simulink model "SINWave"  (R2023a)
settings: Solver=VariableStepAuto  StartTime=0.0  StopTime=10.0  RelTol=1e-3
settings Model: Creator=Lenovo  LastModifiedBy=Lenovo

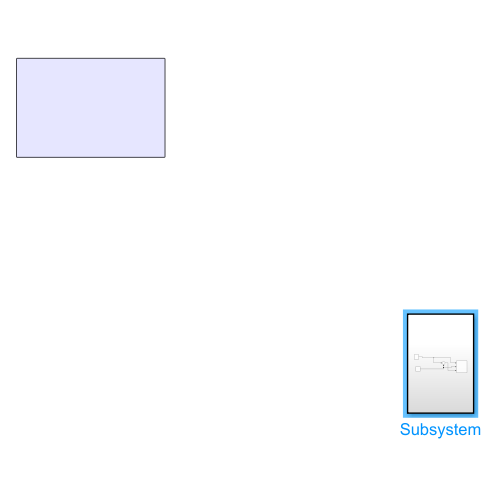
[thumbnail: Simulink's stored preview of the top-level diagram]
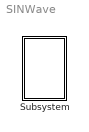
== system SINWave ==
  Subsystem : Subsystem

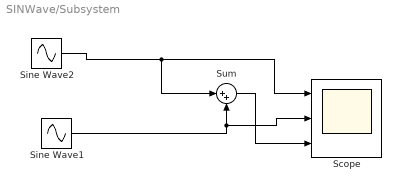
== system SINWave/Subsystem ==
  Scope : Scope  NumInputPorts=3
  Sine Wave1 : Sin  SampleTime=0
  Sine Wave2 : Sin  Amplitude=3  SampleTime=0
  Sum : Sum  Inputs=|++
  wires:
  Sine Wave1/1 -> Scope/2, Sum/2
  Sine Wave2/1 -> Sum/1, Scope/1
  Sum/1 -> Scope/3
